simulink model "FerdyanDannesK_07111440000025"  (R2016a)
settings: Solver=VariableStepAuto  StartTime=0.0  StopTime=50  RelTol=1e-3
libraries: simulink x2, dsparch4 x1, dspinverses x1
settings Model: Creator=Ferdyan Dannes  LastModifiedBy=Ferdyan Dannes

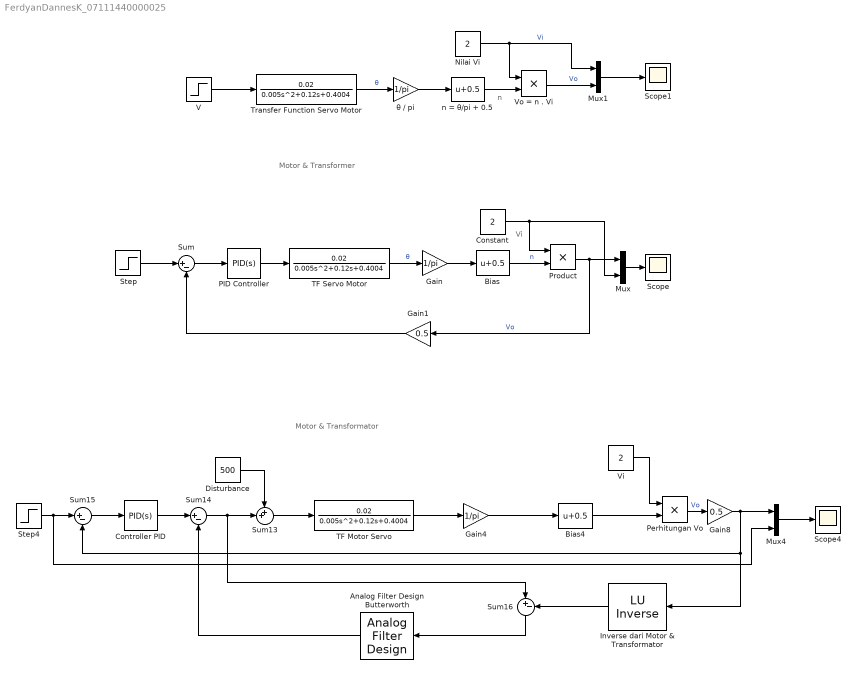
== system FerdyanDannesK_07111440000025 ==
  note: Motor & Transformator
  note: Vi
  note: n
  note: Motor & Transformer
  Analog Filter Design Butterworth : dsparch4/Analog Filter Design  method=Butterworth  filttype=Lowpass  N=3  Wlo=1256.64  Whi=80  Rp=2  Rs=40
  Bias : Bias  Bias=0.5
  Bias4 : Bias  Bias=0.5
  Constant : Constant  Value=2
  Controller PID : simulink/Continuous/PID Controller  Controller=PID  TimeDomain=Continuous-time  SampleTime=-1  IntegratorMethod=Forward Euler  FilterMethod=Forward Euler  Form=Parallel  UseFilter=on  ControllerParametersSource=internal  P=183.934906267807  I=671.812484086527  D=8.27479051060135  N=1119.47712213449  InitialConditionSource=internal  InitialConditionForIntegrator=0  InitialConditionForFilter=0  ExternalReset=none  LimitOutput=off  UpperSaturationLimit=inf  LowerSaturationLimit=-inf  LinearizeAsGain=on  AntiWindupMode=none  Kb=1  TrackingMode=off  Kt=1  PParamMin=[]  PParamMax=[]  IParamMin=[]  IParamMax=[]  DParamMin=[]  DParamMax=[]  NParamMin=[]  NParamMax=[]  KbParamMin=[]  KbParamMax=[]  KtParamMin=[]  KtParamMax=[]  POutMin=[]  POutMax=[]  IOutMin=[]  IOutMax=[]  DOutMin=[]  DOutMax=[]  NOutMin=[]  NOutMax=[]  KbOutMin=[]  KbOutMax=[]  KtOutMin=[]  KtOutMax=[]  IntegratorOutMin=[]  IntegratorOutMax=[]  FilterOutMin=[]  FilterOutMax=[]  SumOutMin=[]  SumOutMax=[]  SumI1OutMin=[]  SumI1OutMax=[]  SumI2OutMin=[]  SumI2OutMax=[]  SumI3OutMin=[]  SumI3OutMax=[]  SumDOutMin=[]  SumDOutMax=[]  SaturationOutMin=[]  SaturationOutMax=[]  IntegratorContinuousStateAttributes=''  IntegratorStateMustResolveToSignalObject=off  IntegratorRTWStateStorageClass=Auto  FilterContinuousStateAttributes=''  FilterStateMustResolveToSignalObject=off  FilterRTWStateStorageClass=Auto  DifferentiatorICPrevScaledInput=0  DifferentiatorOutMin=[]  DifferentiatorOutMax=[]
  Disturbance : Constant  Value=500
  Gain : Gain  Gain=1/pi
  Gain1 : Gain  Gain=0.5
  Gain4 : Gain  Gain=1/pi
  Gain8 : Gain  Gain=0.5
  Inverse dari Motor & Transformator : dspinverses/ LU Inverse
  Mux : Mux  Inputs=2
  Mux1 : Mux  Inputs=2
  Mux4 : Mux  Inputs=2
  Nilai Vi : Constant  Value=2
  PID Controller : simulink/Continuous/PID Controller  Controller=PID  TimeDomain=Continuous-time  SampleTime=-1  IntegratorMethod=Forward Euler  FilterMethod=Forward Euler  Form=Parallel  UseFilter=on  ControllerParametersSource=internal  P=183.934906267807  I=671.812484086527  D=8.27479051060135  N=1119.47712213449  InitialConditionSource=internal  InitialConditionForIntegrator=0  InitialConditionForFilter=0  ExternalReset=none  LimitOutput=off  UpperSaturationLimit=inf  LowerSaturationLimit=-inf  LinearizeAsGain=on  AntiWindupMode=none  Kb=1  TrackingMode=off  Kt=1  PParamMin=[]  PParamMax=[]  IParamMin=[]  IParamMax=[]  DParamMin=[]  DParamMax=[]  NParamMin=[]  NParamMax=[]  KbParamMin=[]  KbParamMax=[]  KtParamMin=[]  KtParamMax=[]  POutMin=[]  POutMax=[]  IOutMin=[]  IOutMax=[]  DOutMin=[]  DOutMax=[]  NOutMin=[]  NOutMax=[]  KbOutMin=[]  KbOutMax=[]  KtOutMin=[]  KtOutMax=[]  IntegratorOutMin=[]  IntegratorOutMax=[]  FilterOutMin=[]  FilterOutMax=[]  SumOutMin=[]  SumOutMax=[]  SumI1OutMin=[]  SumI1OutMax=[]  SumI2OutMin=[]  SumI2OutMax=[]  SumI3OutMin=[]  SumI3OutMax=[]  SumDOutMin=[]  SumDOutMax=[]  SaturationOutMin=[]  SaturationOutMax=[]  IntegratorContinuousStateAttributes=''  IntegratorStateMustResolveToSignalObject=off  IntegratorRTWStateStorageClass=Auto  FilterContinuousStateAttributes=''  FilterStateMustResolveToSignalObject=off  FilterRTWStateStorageClass=Auto  DifferentiatorICPrevScaledInput=0  DifferentiatorOutMin=[]  DifferentiatorOutMax=[]
  Perhitungan Vo : Product
  Product : Product
  Scope : Scope
  Scope1 : Scope
  Scope4 : Scope
  Step : Step  SampleTime=0
  Step4 : Step  SampleTime=0
  Sum{,14..16} (4 alike) : Sum  Inputs=|+-
  Sum13 : Sum  Inputs=++|
  TF Motor Servo : TransferFcn  Numerator=[0.02]  Denominator=[0.005 0.12 0.4004]
  TF Servo Motor : TransferFcn  Numerator=[0.02]  Denominator=[0.005 0.12 0.4004]
  Transfer Function Servo Motor : TransferFcn  Numerator=[0.02]  Denominator=[0.005 0.12 0.4004]
  V : Step  SampleTime=0
  Vi : Constant  Value=2
  Vo = n . Vi : Product
  n = θ/pi + 0.5 : Bias  Bias=0.5
  θ / pi : Gain  Gain=1/pi
  wires:
  Step/1 -> Sum/1
  Sum/1 -> PID Controller/1
  PID Controller/1 -> TF Servo Motor/1
  TF Servo Motor/1 -> Gain/1  "θ"
  Gain/1 -> Bias/1
  Constant/1 -> Product/1, Mux/2
  Bias/1 -> Product/2  "n"
  Mux/1 -> Scope/1
  Product/1 -> Gain1/1, Mux/1  "Vo"
  n = θ/pi + 0.5/1 -> Vo = n . Vi/2
  θ / pi/1 -> n = θ/pi + 0.5/1
  Transfer Function Servo Motor/1 -> θ / pi/1  "θ"
  V/1 -> Transfer Function Servo Motor/1
  Mux1/1 -> Scope1/1
  Vi/1 -> Perhitungan Vo/1
  Bias4/1 -> Perhitungan Vo/2
  Gain4/1 -> Bias4/1
  TF Motor Servo/1 -> Gain4/1
  Controller PID/1 -> Sum14/1
  Sum15/1 -> Controller PID/1
  Step4/1 -> Mux4/2, Sum15/1
  Perhitungan Vo/1 -> Gain8/1  "Vo"
  Sum14/1 -> Sum16/1, Sum13/2
  Inverse dari Motor & Transformator/1 -> Sum16/2
  Mux4/1 -> Scope4/1
  Sum13/1 -> TF Motor Servo/1
  Disturbance/1 -> Sum13/1
  Sum16/1 -> Analog Filter Design Butterworth/1
  Analog Filter Design Butterworth/1 -> Sum14/2
  Vo = n . Vi/1 -> Mux1/2  "Vo"
  Nilai Vi/1 -> Mux1/1, Vo = n . Vi/1  "Vi"
  Gain1/1 -> Sum/2
  Gain8/1 -> Inverse dari Motor & Transformator/1, Sum15/2, Mux4/1
